simulink model "uavControl"  (R2023b)
settings: Solver=ode45  StartTime=0  StopTime=100  RelTol=1e-4
undefined symbols (not defined in the file): b, c, C_D_0, C_D_alpha, C_D_delta_e, C_D_q, C_ell_0, C_ell_beta, C_ell_delta_a, C_ell_delta_r, C_ell_p, C_ell_r, C_L_0, C_L_alpha, C_L_delta_e, C_L_q, C_m_0, C_m_alpha, C_m_delta_e, C_m_q, C_n_0, C_n_beta, C_n_delta_a, C_n_delta_r, C_n_p, C_n_r, C_Y_0, C_Y_beta, C_Y_delta_a, C_Y_delta_r, C_Y_p, C_Y_r, dA, dE, dR, dT, Jx, Jxz, Jy, Jz
libraries: simulink x2, aerolibsim3d x2, sim3dlib x1, shared6dof x1
settings Model: PauseTimes=10  Creator=Victor  LastModifiedBy=Victor
settings DataIOCC: ExternalInput=getinputstruct(report30)  InitialState=getstatestruct(report30)
settings DebuggingCC: MaxConsecutiveZCsMsg=warning

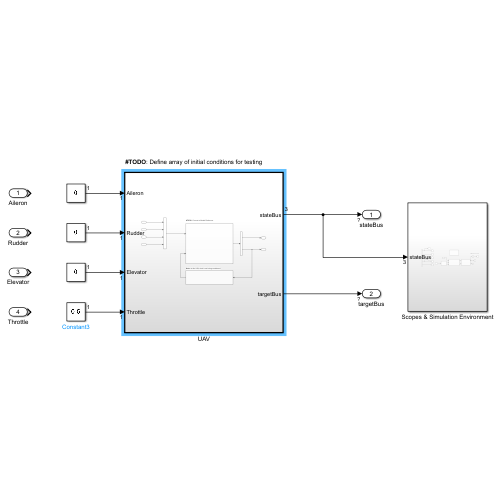
[thumbnail: Simulink's stored preview of the top-level diagram]
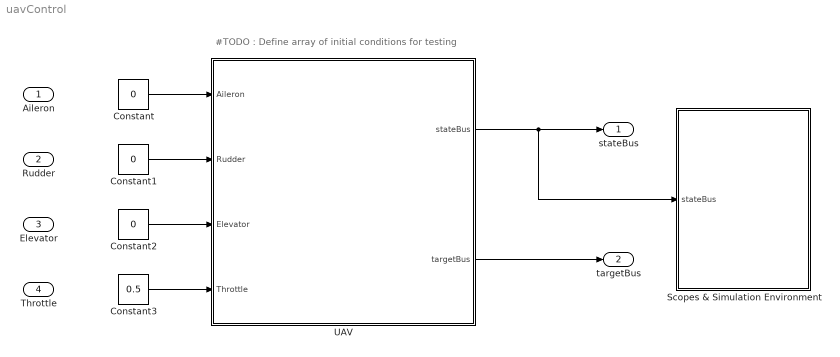
== system uavControl ==
  note: #TODO : Define array of initial conditions for testing
  Aileron : Inport
  Rudder : Inport  Port=2
  Elevator : Inport  Port=3
  Throttle : Inport  Port=4
  Constant : Constant  Value=0
  Constant1 : Constant  Value=0
  Constant2 : Constant  Value=0
  Constant3 : Constant  Value=0.5
  Scopes & Simulation Environment : Subsystem
  UAV : Subsystem  TreatAsAtomicUnit=on
  stateBus : Outport
  targetBus : Outport  Port=2
  wires:
  Constant/1 -> UAV/1(Aileron)
  Constant1/1 -> UAV/2(Rudder)
  Constant2/1 -> UAV/3(Elevator)
  Constant3/1 -> UAV/4(Throttle)
  UAV/2(targetBus) -> targetBus/1
  UAV/1(stateBus) -> Scopes & Simulation Environment/1(stateBus), stateBus/1

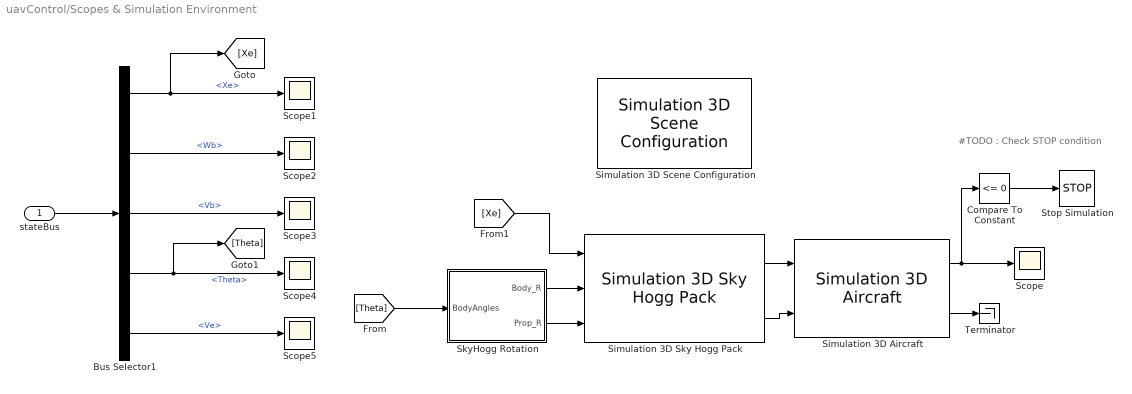
== system uavControl/Scopes & Simulation Environment ==
  note: #TODO : Check STOP condition
  stateBus : Inport
  Bus Selector1 : BusSelector  OutputSignals=Xe,Wb,Vb,Theta,Ve
  Compare To Constant : simulink/Logic and Bit Operations/Compare To Constant  relop=<=  const=0  OutDataTypeStr=boolean
  Scope{,1..5} (6 alike) : Scope
  Simulation 3D Aircraft : aerolibsim3d/Simulation 3D Aircraft  Mesh=Sky Hogg  MeshPath=/MathWorksAerospaceContent/Vehicles/Aircraft/Custom/Mesh/SK_HL20.SK_HL20  MeshPathAT=/MathWorksAerospaceContent/Vehicles/Aircraft/AirTransport/Mesh/SK_AirTransport.SK_AirTransport  MeshPathGA=/MathWorksAerospaceContent/Vehicles/Aircraft/GeneralAviation/Mesh/SK_GeneralAviation.SK_GeneralAviation  AircraftColor=Red  ActorName=SimulinkVehicle1  Translation=[0 0 -2000; zeros(10, 3)]  Rotation=zeros(11, 3)  IsGHSensorEnabled=on  AreGHRaysVisible=off  IsOutputReshapeEnabled=off  GHRayLength=2500  GHBodyOffset=0.90  GHFrontTireRadius=0.21  GHLeftTireRadius=0.21  GHRightTireRadius=0.21  WoWSensorTolerance=0.05  LightsConfig=Automatic lights  LandingLightIntensity=300000  LandingLightConeAngle=15  CustomLeftLandingLightLocation=[0 0 0]  CustomLeftLandingLightOrientation=[0 0 0]  CustomRightLandingLightLocation=[0 0 0]  CustomRightLandingLightOrientation=[0 0 0]  TaxiLightIntensity=150000  TaxiLightConeAngle=36  CustomTaxiLightLocation=[0 0 0]  CustomTaxiLightOrientation=[0 0 0]  NavLightIntensity=500  PositionLightIntensity=500  StrobeLightIntensity=5000  WingtipStrobePeriod=1.5  WingtipStrobePulseWidth=6  TailStrobePeriod=1.5  TailStrobePulseWidth=6  BeaconLightIntensity=4000  BeaconPeriod=1.5  BeaconPulseWidth=10  SampleTime=-1  ActorType=SimulinkVehicle  ID=1  aMode=0  ActorTag=SimulinkVehicle1
  Simulation 3D Scene Configuration : sim3dlib/Simulation 3D Scene Configuration  Priority=0  ProjectFormat=Default Scenes  SceneDesc=Airport  ProjectName=C:\Program Files\MATLAB\R2023b\toolbox\shared\sim3d_projects\automotive_project_windows\UE\WindowsNoEditor\VehicleSimulation.exe  ScenePath=/Game/Maps/HwStrght  EnableOpenDRIVE=off  vehTagList={'Custom';'Scene Origin';'SimulinkVehicle1'}  vehTag=SimulinkVehicle1  FreeCameraInitialTranslation=[0, 0, 0]  FreeCameraDefaultInitialTranslation=[-6, 0, 2]  FreeCameraInitialRotation=[0, 0, 0]  FreeCameraDefaultInitialRotation=[0, -15, 0]  OpVisEn=off  Ts=1/60  EnableWindow=on  EnableRemoteAccess=off  EnableWeather=off  SunAltitude=40.0  SunAzimuth=90  clouds=10  wind=1  fog=0  rain=0  EnableGeospatial=off  OriginHeight=200  OriginLatitude=40.744652  OriginLongitude=-73.988864  MapStyle=Aerial  AdditionalAssetIDs=[]  UseAdvancedSunSky=off  SolarTime=11  TimeZone=-5  Day=21  Month=9  Year=2022  UseDaylightSavingTime=on  DSTStartDay=10  DSTStartMonth=3  DSTEndDay=3  DSTEndMonth=11  DSTSwitchHour=2  sensorTag=MainCamera1  sensorId=1  sensorName=MainCamera1  mountLoc=Origin  offsetFlag=off  tmountOffset=[0, 0, 0]  rmountOffset=[0, 0, 0]  HorizontalResolution=1280  VerticalResolution=720  HorizontalFOV=60  mountPoint=[0 0 0]  mountOrientation=[0 0 0]  aMode=0  ID=1  GeoTrigger=Inactive
      settings: LibrarySourceBlock=aerolibsim3d/Simulation 3D Scene Configuration
  Simulation 3D Sky Hogg Pack : aerolibsim3d/Simulation 3D Sky Hogg Pack  Propeller_R=on  Rudder_R=off  Elevator_R=off  Left_Aileron_R=off  Right_Aileron_R=off  Flaps_R=off  Nose_Wheel_Strut_R=off  Nose_Wheel_R=off  Left_Wheel_R=off  Right_Wheel_R=off  AdjustForCesium=off  Heading0=90
  SkyHogg Rotation : Subsystem
  Stop Simulation : Stop
  Terminator : Terminator
  wires:
  Simulation 3D Sky Hogg Pack/1 -> Simulation 3D Aircraft/1
  SkyHogg Rotation/1(Body_R) -> Simulation 3D Sky Hogg Pack/2
  Simulation 3D Sky Hogg Pack/2 -> Simulation 3D Aircraft/2
  SkyHogg Rotation/2(Prop_R) -> Simulation 3D Sky Hogg Pack/3
  Simulation 3D Aircraft/2 -> Terminator/1
  [Xe] -> Simulation 3D Sky Hogg Pack/1
  [Theta] -> SkyHogg Rotation/1(BodyAngles)
  stateBus/1 -> Bus Selector1/1
  Compare To Constant/1 -> Stop Simulation/1
  Bus Selector1/4 -> Scope4/1, [Theta]  "<Theta>"
  Bus Selector1/1 -> Scope1/1, [Xe]  "<Xe>"
  Bus Selector1/3 -> Scope3/1  "<Vb>"
  Bus Selector1/2 -> Scope2/1  "<Wb>"
  Simulation 3D Aircraft/1 -> Compare To Constant/1, Scope/1
  Bus Selector1/5 -> Scope5/1  "<Ve>"

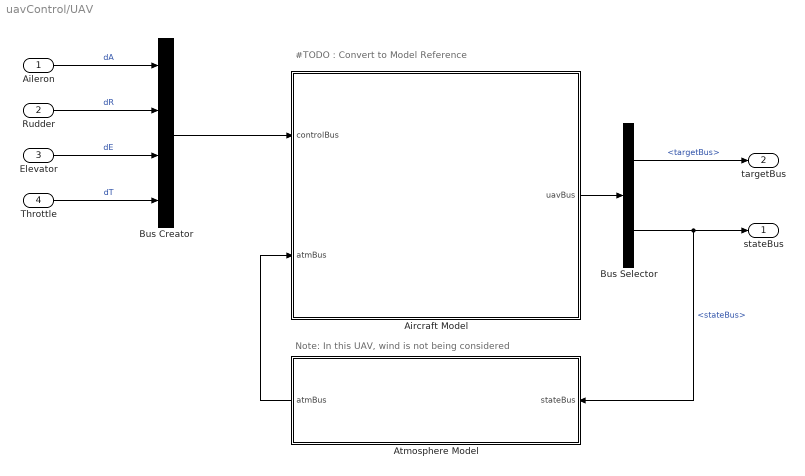
== system uavControl/UAV ==
  note: #TODO : Convert to Model Reference
  note: Note: In this UAV, wind is not being considered
  Aileron : Inport
  Rudder : Inport  Port=2
  Elevator : Inport  Port=3
  Throttle : Inport  Port=4
  Aircraft Model : Subsystem  TreatAsAtomicUnit=on
  Atmosphere Model : Subsystem
  Bus Creator : BusCreator  Inputs=dA,dR,dE,dT
  Bus Selector : BusSelector  OutputSignals=targetBus,stateBus
  stateBus : Outport
  targetBus : Outport  Port=2
  wires:
  Aileron/1 -> Bus Creator/1  "dA"
  Rudder/1 -> Bus Creator/2  "dR"
  Elevator/1 -> Bus Creator/3  "dE"
  Throttle/1 -> Bus Creator/4  "dT"
  Bus Creator/1 -> Aircraft Model/1(controlBus)
  Aircraft Model/1(uavBus) -> Bus Selector/1
  Bus Selector/2 -> Atmosphere Model/1(stateBus), stateBus/1  "<stateBus>"
  Atmosphere Model/1(atmBus) -> Aircraft Model/2(atmBus)
  Bus Selector/1 -> targetBus/1  "<targetBus>"

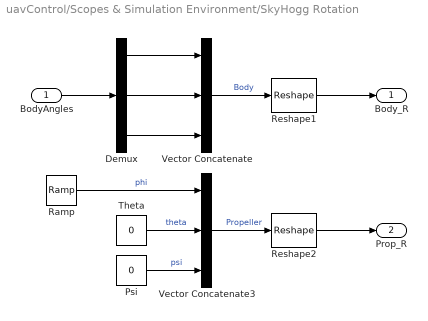
== system uavControl/Scopes & Simulation Environment/SkyHogg Rotation ==
  BodyAngles : Inport
  Demux : Demux  Outputs=3
  Psi : Constant  Value=0
  Ramp : simulink/Sources/Ramp  slope=157  start=0  InitialOutput=0
  Reshape1 : Reshape  OutputDimensionality=Row vector (2-D)
  Reshape2 : Reshape  OutputDimensionality=Row vector (2-D)
  Theta : Constant  Value=0
  Vector Concatenate : Concatenate  NumInputs=3
  Vector Concatenate3 : Concatenate  NumInputs=3
  Body_R : Outport
  Prop_R : Outport  Port=2
  wires:
  Vector Concatenate/1 -> Reshape1/1  "Body"
  Reshape1/1 -> Body_R/1
  Vector Concatenate3/1 -> Reshape2/1  "Propeller"
  Psi/1 -> Vector Concatenate3/3  "psi"
  Theta/1 -> Vector Concatenate3/2  "theta"
  Ramp/1 -> Vector Concatenate3/1  "phi"
  Reshape2/1 -> Prop_R/1
  BodyAngles/1 -> Demux/1
  Demux/1 -> Vector Concatenate/1
  Demux/2 -> Vector Concatenate/2
  Demux/3 -> Vector Concatenate/3

== system uavControl/UAV/Aircraft Model ==
  note: #TODO : Convert to Model Reference
  controlBus : Inport
  atmBus : Inport  Port=2
  Aircraft Dynamics : Subsystem  TreatAsAtomicUnit=on
  Bus Setup : Subsystem
  Equations of Motion : Subsystem
  uavBus : Outport
  wires:
  Aircraft Dynamics/1(forceBus) -> Equations of Motion/1(forceBus)
  controlBus/1 -> Bus Setup/2(controlBus)
  Bus Setup/1(uavBus) -> Aircraft Dynamics/1(uavBus), uavBus/1
  Equations of Motion/1(stateBus) -> Bus Setup/1(stateBus)
  atmBus/1 -> Bus Setup/3(atmBus)

== system uavControl/UAV/Atmosphere Model ==
  stateBus : Inport
  Terminator : Terminator
  Zero : Constant  Value=[0 0 0]
  Out Bus Element : Outport  PortName=atmBus  Element=windSpeed
  wires:
  stateBus/1 -> Terminator/1
  Zero/1 -> Out Bus Element/1

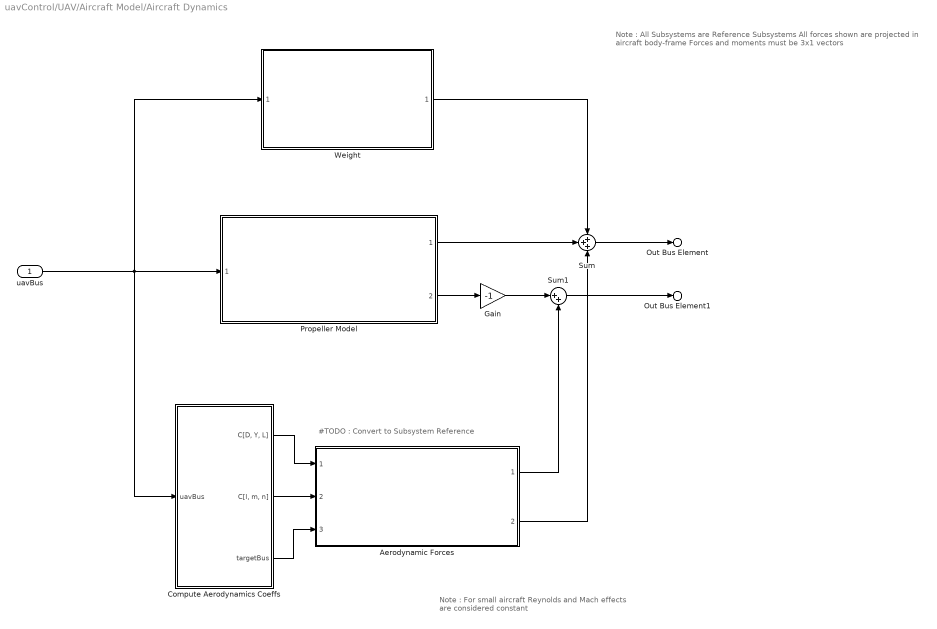
== system uavControl/UAV/Aircraft Model/Aircraft Dynamics ==
  note: Note :
      | All Subsystems are Reference Subsystems
      | All forces shown are projected in aircraft body-frame
      | Forces and moments must be 3x1 vectors
  note: #TODO : Convert to Subsystem Reference
  note: Note : For small aircraft Reynolds and Mach effects are considered constant
  uavBus : Inport
  Aerodynamic Forces : Subsystem  ReferencedSubsystem=aeroForces
  Compute Aerodynamics Coeffs : Subsystem
  Gain : Gain  Gain=-1
  Propeller Model : Subsystem  ReferencedSubsystem=propellerModel
  Sum : Sum  Inputs=+++
  Sum1 : Sum  Inputs=|++
  Weight : Subsystem  ReferencedSubsystem=airframeWeight
  Out Bus Element : Outport  PortName=forceBus  Element=F_b
  Out Bus Element1 : Outport  PortName=forceBus  Element=m_b
  wires:
  Sum/1 -> Out Bus Element/1
  Sum1/1 -> Out Bus Element1/1
  uavBus/1 -> Weight/1, Propeller Model/1, Compute Aerodynamics Coeffs/1(uavBus)
  Weight/1 -> Sum/1
  Propeller Model/2 -> Gain/1
  Propeller Model/1 -> Sum/2
  Gain/1 -> Sum1/1
  Aerodynamic Forces/2 -> Sum/3
  Aerodynamic Forces/1 -> Sum1/2
  Compute Aerodynamics Coeffs/3(targetBus) -> Aerodynamic Forces/3
  Compute Aerodynamics Coeffs/2("C[l, m, n]") -> Aerodynamic Forces/2
  Compute Aerodynamics Coeffs/1("C[D, Y, L]") -> Aerodynamic Forces/1

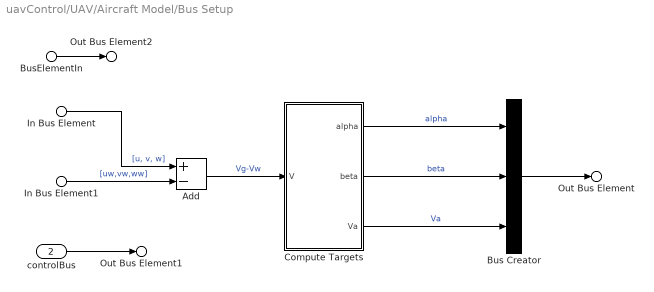
== system uavControl/UAV/Aircraft Model/Bus Setup ==
  BusElementIn : Inport  PortName=stateBus
  In Bus Element : Inport  PortName=stateBus  Element=Vb
  controlBus : Inport  Port=2
  In Bus Element1 : Inport  Port=3  PortName=atmBus  Element=windSpeed
  Add : Sum  Inputs=+-
  Bus Creator : BusCreator  Inputs=3
  Compute Targets : Subsystem
  Out Bus Element1 : Outport  PortName=uavBus  Element=controlBus
  Out Bus Element : Outport  PortName=uavBus  Element=targetBus
  Out Bus Element2 : Outport  PortName=uavBus  Element=stateBus
  wires:
  In Bus Element1/1 -> Add/2  "[uw,vw,ww]"
  In Bus Element/1 -> Add/1  "[u, v, w]"
  Add/1 -> Compute Targets/1(V)  "Vg-Vw"
  Compute Targets/1(alpha) -> Bus Creator/1  "alpha"
  Compute Targets/3(Va) -> Bus Creator/3  "Va"
  Compute Targets/2(beta) -> Bus Creator/2  "beta"
  controlBus/1 -> Out Bus Element1/1
  Bus Creator/1 -> Out Bus Element/1
  BusElementIn/1 -> Out Bus Element2/1

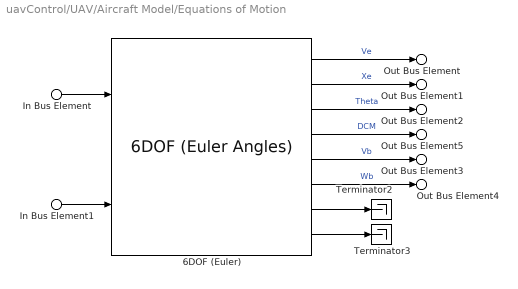
== system uavControl/UAV/Aircraft Model/Equations of Motion ==
  In Bus Element1 : Inport  PortName=forceBus  Element=m_b
  In Bus Element : Inport  PortName=forceBus  Element=F_b
  6DOF (Euler) : shared6dof/6DOF (Euler Angles)  units=Metric (MKS)  mtype=Fixed  rep=Euler Angles  xme_0=x_0  Vm_0=v_0  eul_0=theta_0  pm_0=w_0  mass_0=mass  mass_e=0.5  mass_f=2.0  inertia=[Jx 0 -Jxz; 0 Jy 0; -Jxz 0 Jz]  inertia_e=eye(3)  inertia_f=2*eye(3)  k_quat=1.0  vre_flag=on  abi_flag=off  aMode=0  xme_statename=''  Vm_statename=''  eul_statename=''  quat_statename=''  pm_statename=''  mass_statename=''
      settings: LibrarySourceBlock=aerolib6dof2/6DOF (Quaternion)
  Terminator2 : Terminator
  Terminator3 : Terminator
  Out Bus Element : Outport  PortName=stateBus  Element=Ve
  Out Bus Element1 : Outport  PortName=stateBus  Element=Xe
  Out Bus Element2 : Outport  PortName=stateBus  Element=Theta
  Out Bus Element3 : Outport  PortName=stateBus  Element=Vb
  Out Bus Element4 : Outport  PortName=stateBus  Element=Wb
  Out Bus Element5 : Outport  PortName=stateBus  Element=DCM
  wires:
  6DOF (Euler)/1 -> Out Bus Element/1  "Ve"
  6DOF (Euler)/2 -> Out Bus Element1/1  "Xe"
  6DOF (Euler)/3 -> Out Bus Element2/1  "Theta"
  6DOF (Euler)/6 -> Out Bus Element4/1  "Wb"
  6DOF (Euler)/7 -> Terminator2/1
  6DOF (Euler)/4 -> Out Bus Element5/1  "DCM"
  6DOF (Euler)/5 -> Out Bus Element3/1  "Vb"
  6DOF (Euler)/8 -> Terminator3/1
  In Bus Element/1 -> 6DOF (Euler)/1
  In Bus Element1/1 -> 6DOF (Euler)/2

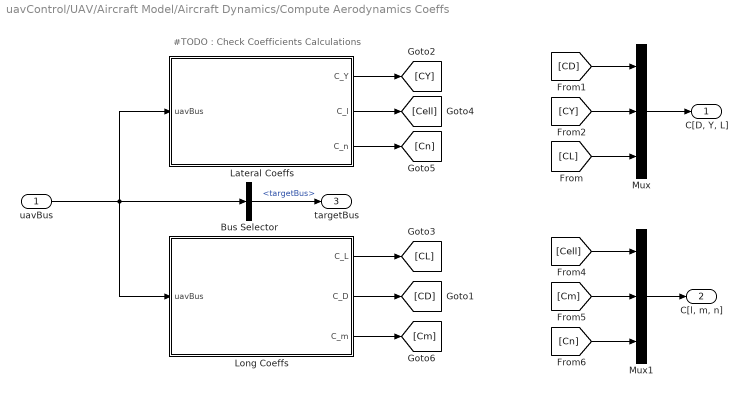
== system uavControl/UAV/Aircraft Model/Aircraft Dynamics/Compute Aerodynamics Coeffs ==
  note: #TODO : Check Coefficients Calculations
  uavBus : Inport
  Bus Selector : BusSelector  OutputSignals=targetBus
  Lateral Coeffs : Subsystem
  Long Coeffs : Subsystem
  Mux : Mux  Inputs=3
  Mux1 : Mux  Inputs=3
  "C[D, Y, L]" : Outport
  "C[l, m, n]" : Outport  Port=2
  targetBus : Outport  Port=3
  wires:
  uavBus/1 -> Long Coeffs/1(uavBus), Lateral Coeffs/1(uavBus), Bus Selector/1
  Mux/1 -> "C[D, Y, L]"/1
  Bus Selector/1 -> targetBus/1  "<targetBus>"
  Long Coeffs/2(C_D) -> [CD]
  Lateral Coeffs/1(C_Y) -> [CY]
  Long Coeffs/1(C_L) -> [CL]
  [CD] -> Mux/1
  [CY] -> Mux/2
  [CL] -> Mux/3
  [Cn] -> Mux1/3
  Mux1/1 -> "C[l, m, n]"/1
  [Cm] -> Mux1/2
  [Cell] -> Mux1/1
  Lateral Coeffs/2(C_l) -> [Cell]
  Lateral Coeffs/3(C_n) -> [Cn]
  Long Coeffs/3(C_m) -> [Cm]

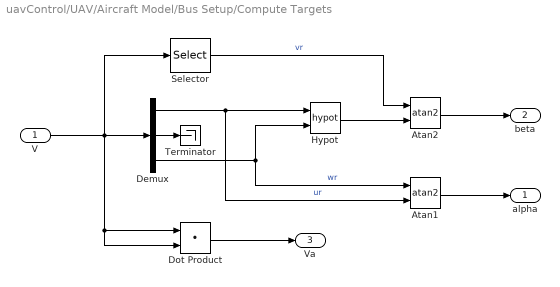
== system uavControl/UAV/Aircraft Model/Bus Setup/Compute Targets ==
  V : Inport
  Atan1 : Trigonometry  Operator=atan2
  Atan2 : Trigonometry  Operator=atan2
  Demux : Demux  Outputs=3
  Dot Product : DotProduct  OutDataTypeStr=Inherit: Inherit via internal rule
  Hypot : Math  Operator=hypot
  Selector : Selector  InputPortWidth=3  IndexOptions=Index vector (dialog)  Indices=[2]  OutputSizes=1
  Terminator : Terminator
  alpha : Outport
  beta : Outport  Port=2
  Va : Outport  Port=3
  wires:
  V/1 -> Dot Product/1, Dot Product/2, Demux/1, Selector/1
  Dot Product/1 -> Va/1
  Hypot/1 -> Atan2/2
  Atan2/1 -> beta/1
  Selector/1 -> Atan2/1  "vr"
  Atan1/1 -> alpha/1
  Demux/3 -> Hypot/2, Atan1/1  "wr"
  Demux/1 -> Atan1/2, Hypot/1  "ur"
  Demux/2 -> Terminator/1

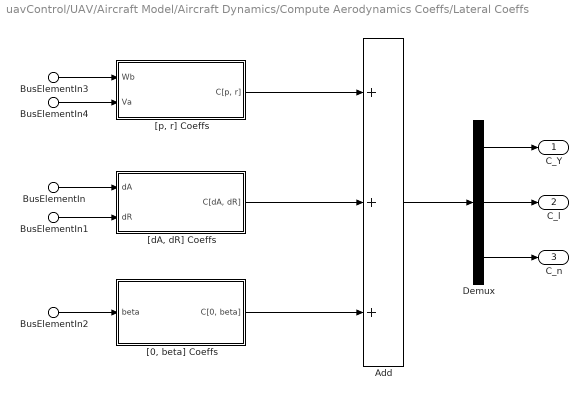
== system uavControl/UAV/Aircraft Model/Aircraft Dynamics/Compute Aerodynamics Coeffs/Lateral Coeffs ==
  BusElementIn3 : Inport  PortName=uavBus  Element=stateBus.Wb
  BusElementIn : Inport  PortName=uavBus  Element=controlBus.dA
  BusElementIn1 : Inport  PortName=uavBus  Element=controlBus.dR
  BusElementIn2 : Inport  PortName=uavBus  Element=targetBus.beta
  BusElementIn4 : Inport  PortName=uavBus  Element=targetBus.Va
  Add : Sum  Inputs=+++
  Demux : Demux  Outputs=3
  "[0, beta] Coeffs" : Subsystem
  "[dA, dR] Coeffs" : Subsystem
  "[p, r] Coeffs" : Subsystem
  C_Y : Outport
  C_l : Outport  Port=2
  C_n : Outport  Port=3
  wires:
  BusElementIn3/1 -> "[p, r] Coeffs"/1(Wb)
  BusElementIn4/1 -> "[p, r] Coeffs"/2(Va)
  BusElementIn/1 -> "[dA, dR] Coeffs"/1(dA)
  BusElementIn1/1 -> "[dA, dR] Coeffs"/2(dR)
  BusElementIn2/1 -> "[0, beta] Coeffs"/1(beta)
  "[p, r] Coeffs"/1("C[p, r]") -> Add/1
  "[dA, dR] Coeffs"/1("C[dA, dR]") -> Add/2
  "[0, beta] Coeffs"/1("C[0, beta]") -> Add/3
  Add/1 -> Demux/1
  Demux/1 -> C_Y/1
  Demux/2 -> C_l/1
  Demux/3 -> C_n/1

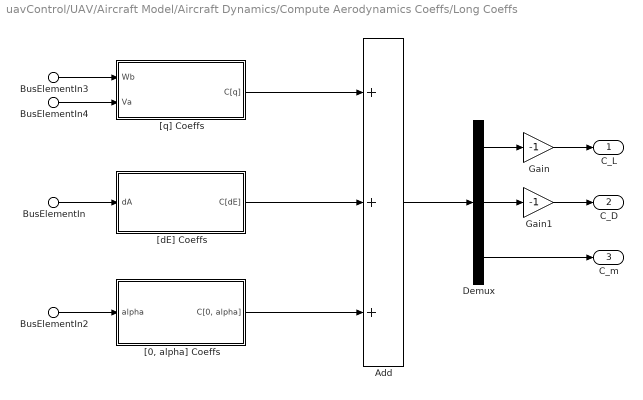
== system uavControl/UAV/Aircraft Model/Aircraft Dynamics/Compute Aerodynamics Coeffs/Long Coeffs ==
  BusElementIn3 : Inport  PortName=uavBus  Element=stateBus.Wb
  BusElementIn : Inport  PortName=uavBus  Element=controlBus.dE
  BusElementIn2 : Inport  PortName=uavBus  Element=targetBus.alpha
  BusElementIn4 : Inport  PortName=uavBus  Element=targetBus.Va
  Add : Sum  Inputs=+++
  Demux : Demux  Outputs=3
  Gain : Gain  Gain=-1
  Gain1 : Gain  Gain=-1
  "[0, alpha] Coeffs" : Subsystem
  "[dE] Coeffs" : Subsystem
  "[q] Coeffs" : Subsystem
  C_L : Outport
  C_D : Outport  Port=2
  C_m : Outport  Port=3
  wires:
  BusElementIn3/1 -> "[q] Coeffs"/1(Wb)
  BusElementIn/1 -> "[dE] Coeffs"/1(dA)
  Add/1 -> Demux/1
  "[dE] Coeffs"/1(C[dE]) -> Add/2
  BusElementIn4/1 -> "[q] Coeffs"/2(Va)
  "[q] Coeffs"/1(C[q]) -> Add/1
  "[0, alpha] Coeffs"/1("C[0, alpha]") -> Add/3
  BusElementIn2/1 -> "[0, alpha] Coeffs"/1(alpha)
  Demux/1 -> Gain/1
  Demux/2 -> Gain1/1
  Demux/3 -> C_m/1
  Gain/1 -> C_L/1
  Gain1/1 -> C_D/1

== system uavControl/UAV/Aircraft Model/Aircraft Dynamics/Compute Aerodynamics Coeffs/Lateral Coeffs/[0, beta] Coeffs ==
  beta : Inport
  Add : Sum
  C[0] : Constant  Value=[C_Y_0, C_ell_0, C_n_0]
  C[beta] : Constant  Value=[C_Y_beta C_ell_beta, C_n_beta]
  Product : Product
  "C[0, beta]" : Outport
  wires:
  beta/1 -> Product/2
  C[beta]/1 -> Product/1
  Product/1 -> Add/1
  C[0]/1 -> Add/2
  Add/1 -> "C[0, beta]"/1

== system uavControl/UAV/Aircraft Model/Aircraft Dynamics/Compute Aerodynamics Coeffs/Lateral Coeffs/[dA, dR] Coeffs ==
  dA : Inport
  dR : Inport  Port=2
  Add : Sum
  C[deltaA] : Constant  Value=[C_Y_delta_a, C_ell_delta_a, C_n_delta_a]
  C[deltaR] : Constant  Value=[C_Y_delta_r, C_ell_delta_r, C_n_delta_r]
  Product : Product
  Product1 : Product
  "C[dA, dR]" : Outport
  wires:
  dA/1 -> Product/2
  C[deltaA]/1 -> Product/1
  dR/1 -> Product1/1
  C[deltaR]/1 -> Product1/2
  Product/1 -> Add/1
  Product1/1 -> Add/2
  Add/1 -> "C[dA, dR]"/1

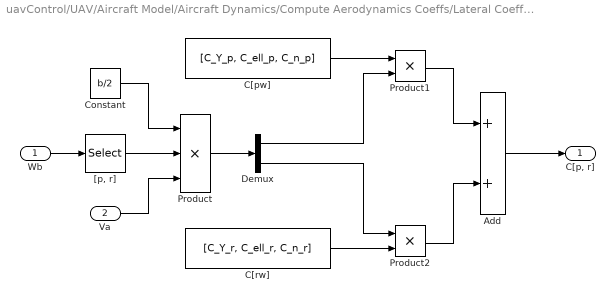
== system uavControl/UAV/Aircraft Model/Aircraft Dynamics/Compute Aerodynamics Coeffs/Lateral Coeffs/[p, r] Coeffs ==
  Wb : Inport
  Va : Inport  Port=2
  Add : Sum
  C[pw] : Constant  Value=[C_Y_p, C_ell_p, C_n_p]
  C[rw] : Constant  Value=[C_Y_r, C_ell_r, C_n_r]
  Constant : Constant  Value=b/2
  Demux : Demux  Outputs=2
  Product : Product  Inputs=3
  Product1 : Product
  Product2 : Product
  "[p, r]" : Selector  InputPortWidth=3  IndexOptions=Index vector (dialog)  Indices=[1 3]  OutputSizes=1
  "C[p, r]" : Outport
  wires:
  Wb/1 -> "[p, r]"/1
  "[p, r]"/1 -> Product/2
  Va/1 -> Product/3
  Constant/1 -> Product/1
  Product/1 -> Demux/1
  C[pw]/1 -> Product1/1
  Demux/1 -> Product1/2
  Demux/2 -> Product2/1
  C[rw]/1 -> Product2/2
  Product1/1 -> Add/1
  Product2/1 -> Add/2
  Add/1 -> "C[p, r]"/1

== system uavControl/UAV/Aircraft Model/Aircraft Dynamics/Compute Aerodynamics Coeffs/Long Coeffs/[0, alpha] Coeffs ==
  alpha : Inport
  Add : Sum
  C[0] : Constant  Value=[C_L_0, C_D_0, C_m_0]
  C[alpha] : Constant  Value=[C_L_alpha C_D_alpha, C_m_alpha]
  Product : Product
  "C[0, alpha]" : Outport
  wires:
  alpha/1 -> Product/2
  C[alpha]/1 -> Product/1
  Product/1 -> Add/1
  C[0]/1 -> Add/2
  Add/1 -> "C[0, alpha]"/1

== system uavControl/UAV/Aircraft Model/Aircraft Dynamics/Compute Aerodynamics Coeffs/Long Coeffs/[dE] Coeffs ==
  dA : Inport
  C[deltaE] : Constant  Value=[C_L_delta_e, C_D_delta_e, C_m_delta_e]
  Product : Product
  C[dE] : Outport
  wires:
  dA/1 -> Product/2
  C[deltaE]/1 -> Product/1
  Product/1 -> C[dE]/1

== system uavControl/UAV/Aircraft Model/Aircraft Dynamics/Compute Aerodynamics Coeffs/Long Coeffs/[q] Coeffs ==
  Wb : Inport
  Va : Inport  Port=2
  C[qw] : Constant  Value=[C_L_q, C_D_q, C_m_q]
  Constant : Constant  Value=c/2
  Product : Product  Inputs=3
  Product1 : Product
  "[q]" : Selector  InputPortWidth=3  IndexOptions=Index vector (dialog)  Indices=[2]  OutputSizes=1
  C[q] : Outport
  wires:
  Wb/1 -> "[q]"/1
  "[q]"/1 -> Product/2
  Va/1 -> Product/3
  Constant/1 -> Product/1
  Product/1 -> Product1/2
  C[qw]/1 -> Product1/1
  Product1/1 -> C[q]/1
